simulink model "TEST3_Control_Simulink"  (R2025b)
settings: Solver=ode3  StartTime=0.0  StopTime=500  FixedStep=0.1  RelTol=1e-3
libraries: slpidlib x2
settings Model: Creator=daniel.camacho  LastModifiedBy=daniel.camacho

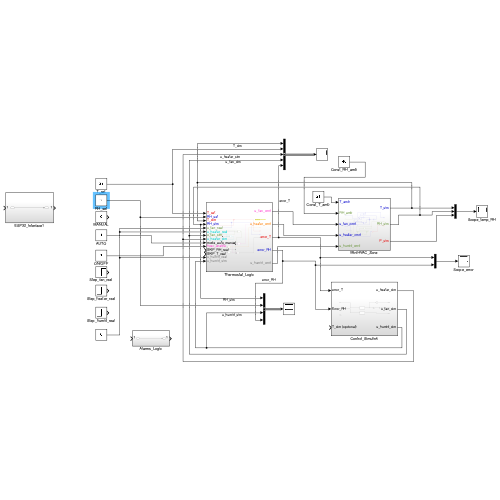
[thumbnail: Simulink's stored preview of the top-level diagram]
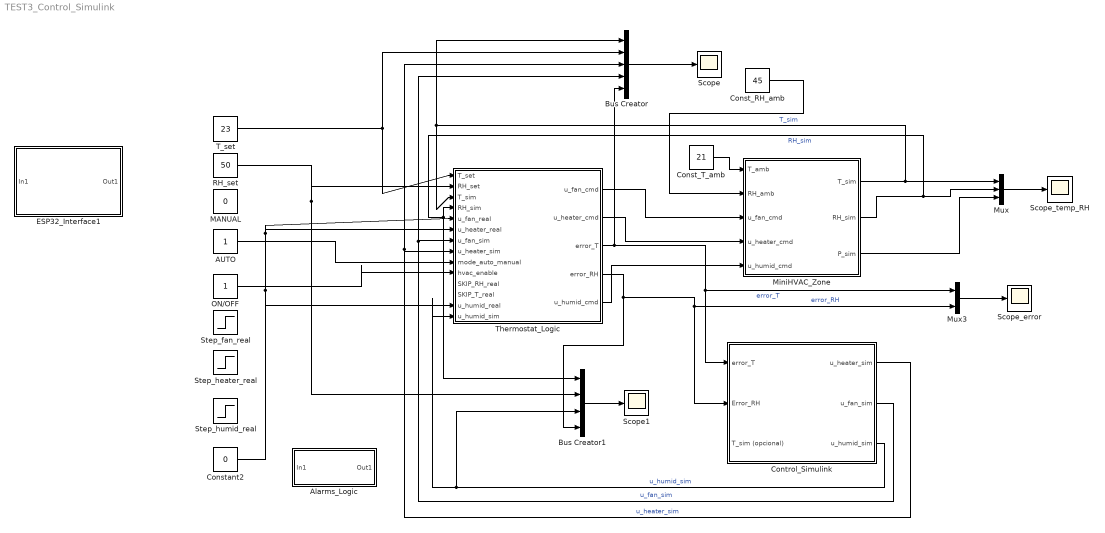
== system TEST3_Control_Simulink ==
  AUTO : Constant
  Alarms_Logic : Subsystem
  Bus Creator : BusCreator  Inputs=5
  Bus Creator1 : BusCreator  Inputs=4
  Const_RH_amb : Constant  Value=45
  Const_T_amb : Constant  Value=21
  Constant2 : Constant  Value=0
  Control_Simulink : Subsystem
  ESP32_Interface1 : Subsystem
  MANUAL : Constant  Value=0
  MiniHVAC_Zone : Subsystem
  Mux : Mux  Inputs=3
  Mux3 : Mux  Inputs=2
  ON/OFF : Constant
  RH_set : Constant  Value=50
  Scope : Scope
      settings: ActiveDisplayYMinimum=-7.8749999999999991  ActiveDisplayYMaximum=30.875  DataLoggingVariableName=ScopeData2
  Scope1 : Scope
      settings: ActiveDisplayYMinimum=-3.7726610995942522  ActiveDisplayYMaximum=85.751334887185152
  Scope_error : Scope
      settings: ActiveDisplayYMinimum=-12.97347055879947  ActiveDisplayYMaximum=6.9970522843110521  DataLoggingVariableName=ScopeData4
  Scope_temp_RH : Scope
      settings: ActiveDisplayYMinimum=-1  ActiveDisplayYMaximum=1
  Step_fan_real : Step  Time=10  SampleTime=0
  Step_heater_real : Step  Time=20  SampleTime=0
  Step_humid_real : Step  Time=10  SampleTime=0
  T_set : Constant  Value=23
  Thermostat_Logic : Subsystem
  wires:
  RH_set/1 -> Thermostat_Logic/2(RH_set), Bus Creator1/2
  ON/OFF/1 -> Thermostat_Logic/10(hvac_enable)
  Constant2/1 -> Thermostat_Logic/13(u_humid_real), Thermostat_Logic/6(u_heater_real), Thermostat_Logic/5(u_fan_real)
  MiniHVAC_Zone/2(RH_sim) -> Mux/2, Bus Creator1/1, Thermostat_Logic/4(RH_sim)  "RH_sim"
  Thermostat_Logic/1(u_fan_cmd) -> MiniHVAC_Zone/3(u_fan_cmd)
  Thermostat_Logic/2(u_heater_cmd) -> MiniHVAC_Zone/4(u_heater_cmd)
  Const_T_amb/1 -> MiniHVAC_Zone/1(T_amb)
  Const_RH_amb/1 -> MiniHVAC_Zone/2(RH_amb)
  Mux/1 -> Scope_temp_RH/1
  MiniHVAC_Zone/3(P_sim) -> Mux/3
  Mux3/1 -> Scope_error/1
  Thermostat_Logic/4(error_RH) -> Bus Creator1/4, Mux3/2, Control_Simulink/2(Error_RH)  "error_RH"
  Thermostat_Logic/5(u_humid_cmd) -> MiniHVAC_Zone/5(u_humid_cmd)
  T_set/1 -> Thermostat_Logic/1(T_set), Bus Creator/2
  Thermostat_Logic/3(error_T) -> Mux3/1, Control_Simulink/1(error_T), Bus Creator/5  "error_T"
  MiniHVAC_Zone/1(T_sim) -> Mux/1, Bus Creator/1, Thermostat_Logic/3(T_sim)  "T_sim"
  Control_Simulink/2(u_fan_sim) -> Bus Creator/4, Thermostat_Logic/7(u_fan_sim)  "u_fan_sim"
  Control_Simulink/1(u_heater_sim) -> Bus Creator/3, Thermostat_Logic/8(u_heater_sim)  "u_heater_sim"
  Bus Creator/1 -> Scope/1
  AUTO/1 -> Thermostat_Logic/9(mode_auto_manual)
  Bus Creator1/1 -> Scope1/1
  Control_Simulink/3(u_humid_sim) -> Bus Creator1/3, Thermostat_Logic/14(u_humid_sim)  "u_humid_sim"

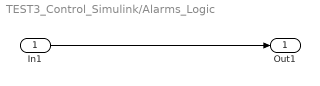
== system TEST3_Control_Simulink/Alarms_Logic ==
  In1 : Inport
  Out1 : Outport
  wires:
  In1/1 -> Out1/1

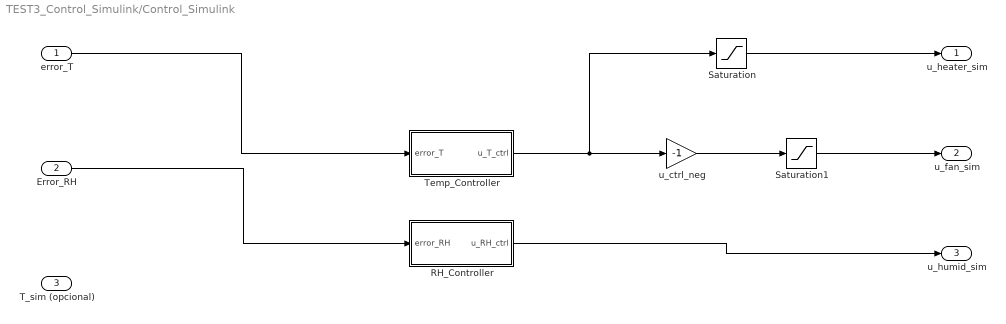
== system TEST3_Control_Simulink/Control_Simulink ==
  error_T : Inport
  Error_RH : Inport  Port=2
  T_sim (opcional) : Inport  Port=3
  RH_Controller : Subsystem
  Saturation : Saturate  UpperLimit=1  LowerLimit=0
  Saturation1 : Saturate  UpperLimit=1  LowerLimit=0
  Temp_Controller : Subsystem
  u_ctrl_neg : Gain  Gain=-1
  u_heater_sim : Outport
  u_fan_sim : Outport  Port=2
  u_humid_sim : Outport  Port=3
  wires:
  Temp_Controller/1(u_T_ctrl) -> u_ctrl_neg/1, Saturation/1
  Saturation/1 -> u_heater_sim/1
  u_ctrl_neg/1 -> Saturation1/1
  Saturation1/1 -> u_fan_sim/1
  error_T/1 -> Temp_Controller/1(error_T)
  Error_RH/1 -> RH_Controller/1(error_RH)
  RH_Controller/1(u_RH_ctrl) -> u_humid_sim/1

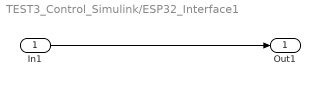
== system TEST3_Control_Simulink/ESP32_Interface1 ==
  In1 : Inport
  Out1 : Outport
  wires:
  In1/1 -> Out1/1

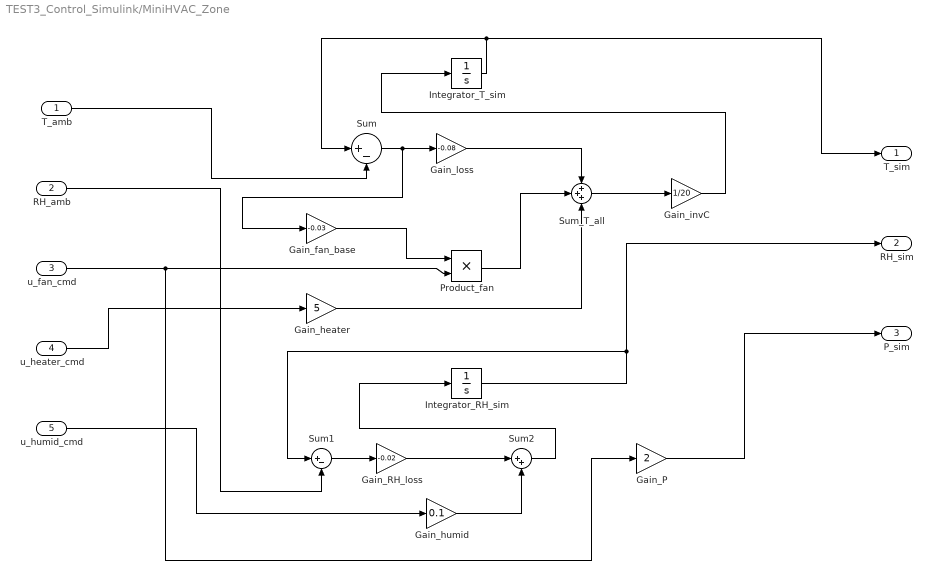
== system TEST3_Control_Simulink/MiniHVAC_Zone ==
  T_amb : Inport
  RH_amb : Inport  Port=2
  u_fan_cmd : Inport  Port=3
  u_heater_cmd : Inport  Port=4
  u_humid_cmd : Inport  Port=5
  Gain_P : Gain  Gain=2
  Gain_RH_loss : Gain  Gain=-0.02
  Gain_fan_base : Gain  Gain=-0.03
  Gain_heater : Gain  Gain=5
  Gain_humid : Gain  Gain=0.1
  Gain_invC : Gain  Gain=1/20
  Gain_loss : Gain  Gain=-0.08
  Integrator_RH_sim : Integrator  InitialCondition=45
  Integrator_T_sim : Integrator  InitialCondition=27
  Product_fan : Product
  Sum : Sum  Inputs=|+-
  Sum1 : Sum  Inputs=|+-
  Sum2 : Sum  Inputs=|++
  Sum_T_all : Sum  Inputs=+++
  T_sim : Outport
  RH_sim : Outport  Port=2
  P_sim : Outport  Port=3
  wires:
  Integrator_T_sim/1 -> T_sim/1, Sum/1
  T_amb/1 -> Sum/2
  Gain_fan_base/1 -> Product_fan/1
  u_fan_cmd/1 -> Gain_P/1, Product_fan/2
  u_heater_cmd/1 -> Gain_heater/1
  Sum/1 -> Gain_loss/1, Gain_fan_base/1
  Gain_loss/1 -> Sum_T_all/1
  Product_fan/1 -> Sum_T_all/2
  Gain_heater/1 -> Sum_T_all/3
  Sum_T_all/1 -> Gain_invC/1
  Gain_invC/1 -> Integrator_T_sim/1
  Integrator_RH_sim/1 -> RH_sim/1, Sum1/1
  RH_amb/1 -> Sum1/2
  Sum1/1 -> Gain_RH_loss/1
  u_humid_cmd/1 -> Gain_humid/1
  Gain_RH_loss/1 -> Sum2/1
  Gain_humid/1 -> Sum2/2
  Sum2/1 -> Integrator_RH_sim/1
  Gain_P/1 -> P_sim/1

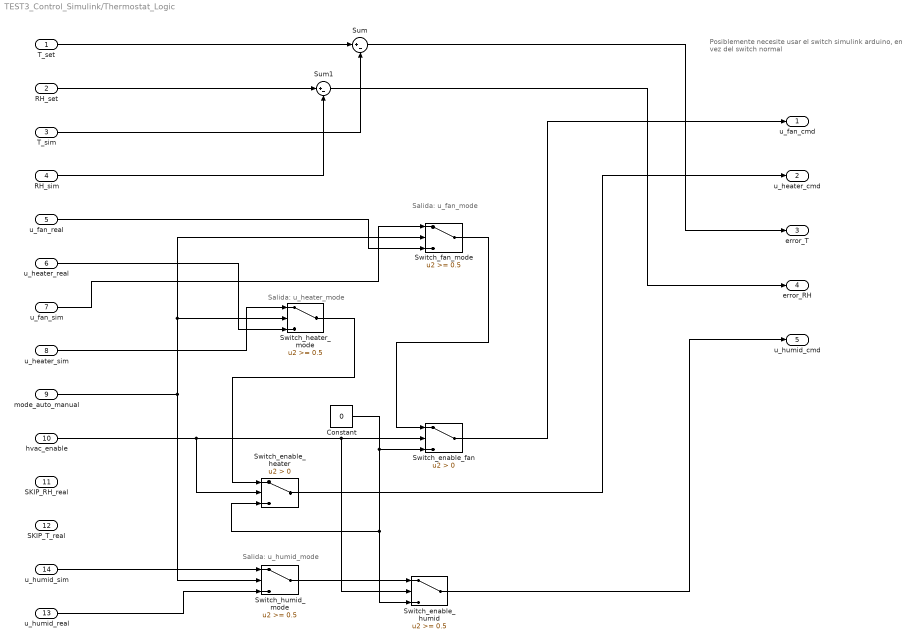
== system TEST3_Control_Simulink/Thermostat_Logic ==
  note: Salida: u_fan_mode
  note: Posiblemente necesite usar el switch simulink arduino,
      | en vez del switch normal
  note: Salida: u_heater_mode
  note: Salida: u_humid_mode
  T_set : Inport
  RH_set : Inport  Port=2
  T_sim : Inport  Port=3
  RH_sim : Inport  Port=4
  u_fan_real : Inport  Port=5
  u_heater_real : Inport  Port=6
  u_fan_sim : Inport  Port=7
  u_heater_sim : Inport  Port=8
  mode_auto_manual : Inport  Port=9
  hvac_enable : Inport  Port=10
  SKIP_RH_real : Inport  Port=11
  SKIP_T_real : Inport  Port=12
  u_humid_real : Inport  Port=13
  u_humid_sim : Inport  Port=14
  Constant : Constant  Value=0
  Sum : Sum  Inputs=|+-
  Sum1 : Sum  Inputs=|+-
  Switch_enable_fan : Switch  Criteria=u2 > Threshold  SaturateOnIntegerOverflow=off  InputSameDT=off
  Switch_enable_heater : Switch  Criteria=u2 > Threshold  SaturateOnIntegerOverflow=off  InputSameDT=off
  Switch_enable_humid : Switch  Threshold=0.5  SaturateOnIntegerOverflow=off  InputSameDT=off
  Switch_fan_mode : Switch  Threshold=0.5  SaturateOnIntegerOverflow=off  InputSameDT=off
  Switch_heater_mode : Switch  Threshold=0.5  OutMin=0  OutMax=1  SaturateOnIntegerOverflow=off  InputSameDT=off
  Switch_humid_mode : Switch  Threshold=0.5  SaturateOnIntegerOverflow=off  InputSameDT=off
  u_fan_cmd : Outport
  u_heater_cmd : Outport  Port=2
  error_T : Outport  Port=3
  error_RH : Outport  Port=4
  u_humid_cmd : Outport  Port=5
  wires:
  T_set/1 -> Sum/1
  T_sim/1 -> Sum/2
  Sum/1 -> error_T/1
  RH_set/1 -> Sum1/1
  RH_sim/1 -> Sum1/2
  Sum1/1 -> error_RH/1
  mode_auto_manual/1 -> Switch_heater_mode/2, Switch_fan_mode/2, Switch_humid_mode/2
  Constant/1 -> Switch_enable_fan/3, Switch_enable_humid/3, Switch_enable_heater/3
  hvac_enable/1 -> Switch_enable_fan/2, Switch_enable_humid/2, Switch_enable_heater/2
  Switch_enable_fan/1 -> u_fan_cmd/1
  Switch_enable_heater/1 -> u_heater_cmd/1
  u_fan_real/1 -> Switch_fan_mode/3
  u_fan_sim/1 -> Switch_fan_mode/1
  u_heater_sim/1 -> Switch_heater_mode/1
  u_heater_real/1 -> Switch_heater_mode/3
  Switch_fan_mode/1 -> Switch_enable_fan/1
  Switch_heater_mode/1 -> Switch_enable_heater/1
  u_humid_sim/1 -> Switch_humid_mode/1
  u_humid_real/1 -> Switch_humid_mode/3
  Switch_humid_mode/1 -> Switch_enable_humid/1
  Switch_enable_humid/1 -> u_humid_cmd/1

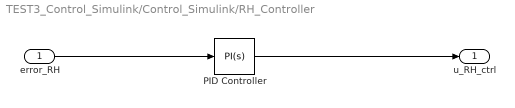
== system TEST3_Control_Simulink/Control_Simulink/RH_Controller ==
  error_RH : Inport
  PID Controller : slpidlib/PID Controller  Controller=PI  Form=Parallel  TimeDomain=Continuous-time  UseExternalTs=off  SampleTime=-1  IntegratorMethod=Forward Euler  FilterMethod=Forward Euler  ControllerParametersSource=internal  P=0.5  I=0.01  UseKiTs=off  D=0  UseExternalDerivativeSource=off  N=100  UseFilter=on  TunerSelectOption=Transfer Function Based (PID Tuner App)  InitialConditionSource=internal  InitialConditionForIntegrator=0  InitialConditionForFilter=0  DifferentiatorICPrevScaledInput=0  ExternalReset=none  TrackingMode=off  Kt=1  LimitOutput=on  SatLimitsSource=internal  UpperSaturationLimit=1  LowerSaturationLimit=0  LinearizeAsGain=on  AntiWindupMode=back-calculation  Kb=1  LimitIntegrator=off  UpperIntegratorSaturationLimit=inf  LowerIntegratorSaturationLimit=-inf  POutMin=[]  POutMax=[]  IOutMin=[]  IOutMax=[]  DOutMin=[]  DOutMax=[]  NOutMin=[]  NOutMax=[]  SumOutMin=[]  SumOutMax=[]  SaturationOutMin=[]  SaturationOutMax=[]  PParamMin=[]  PParamMax=[]  IParamMin=[]  IParamMax=[]  DParamMin=[]  DParamMax=[]  NParamMin=[]  NParamMax=[]  KbParamMin=[]  KbParamMax=[]  KtParamMin=[]  KtParamMax=[]  KbOutMin=[]  KbOutMax=[]  KtOutMin=[]  KtOutMax=[]  IntegratorOutMin=[]  IntegratorOutMax=[]  FilterOutMin=[]  FilterOutMax=[]  SumI1OutMin=[]  SumI1OutMax=[]  SumI2OutMin=[]  SumI2OutMax=[]  SumI3OutMin=[]  SumI3OutMax=[]  SumI4OutMin=[]  SumI4OutMax=[]  SumDOutMin=[]  SumDOutMax=[]  DifferentiatorOutMin=[]  DifferentiatorOutMax=[]  FilterDiffOutCoefMin=[]  FilterDiffOutCoefMax=[]  ReciprocalOutMin=[]  ReciprocalOutMax=[]  SumDenOutMin=[]  SumDenOutMax=[]  SumNumOutMin=[]  SumNumOutMax=[]  DivideOutMin=[]  DivideOutMax=[]  UdiffTsProdOutMin=[]  UdiffTsProdOutMax=[]  NTsProdOutMin=[]  NTsProdOutMax=[]  UintegralTsProdOutMin=[]  UintegralTsProdOutMax=[]  UngainTsProdOutMin=[]  UngainTsProdOutMax=[]  ClampingZeroOutDataTypeStr=Inherit: Inherit via back propagation  ClampingZeroOutMin=[]  ClampingZeroOutMax=[]  FilterDenConstantOutDataTypeStr=Inherit: Inherit via back propagation  FilterDenConstantOutMin=[]  FilterDenConstantOutMax=[]  PCopyOutDataTypeStr=Inherit: Inherit via back propagation  PCopyOutMin=[]  PCopyOutMax=[]  NCopyOutDataTypeStr=Inherit: Inherit via back propagation  NCopyOutMin=[]  NCopyOutMax=[]  IntegratorContinuousStateAttributes=''  IntegratorStateMustResolveToSignalObject=off  IntegratorRTWStateStorageClass=Auto  FilterContinuousStateAttributes=''  FilterStateMustResolveToSignalObject=off  FilterRTWStateStorageClass=Auto  ParallelPVariant=InternalParameters  IdealPVariant=Disabled  IVariant=InternalParameters  DVariant=Disabled  IntegratorVariant=Continuous  SatVariant=Enabled  AWVariant=BackCalculation  PCopyVariant=Disabled  TRVariant=Disabled  FdbkBlocksVariant=Forward  IdealPFdbkVariant=Disabled  SatFdbkVariant=Disabled  DerivativeFilterVariant=Disabled  NVariant=Disabled  NCopyVariant=Disabled_SignalSpec  FilterICVariant=Disabled  IntegratorICVariant=InternalICs  ExternalResetVariant=Disabled  TRSumVariant=Passthrough  SumFdbkVariant=Disabled  SumVariant=Sum_PI  TsampFilterVariant=InternalTs  TsampNgainVariant=Passthrough  TsampIntegralVariant=Disabled_SignalSpec  ExternalSaturationOutDataTypeStr=Inherit: Same as second input  DerivativeSourceVariant=Disabled  PreIntVariant=InternalPreInt
  u_RH_ctrl : Outport
  wires:
  error_RH/1 -> PID Controller/1
  PID Controller/1 -> u_RH_ctrl/1

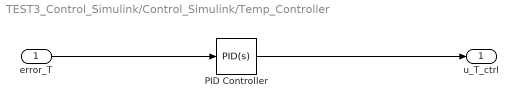
== system TEST3_Control_Simulink/Control_Simulink/Temp_Controller ==
  error_T : Inport
  PID Controller : slpidlib/PID Controller  Controller=PID  Form=Parallel  TimeDomain=Continuous-time  UseExternalTs=off  SampleTime=-1  IntegratorMethod=Forward Euler  FilterMethod=Forward Euler  ControllerParametersSource=internal  P=0.5  I=0.01  UseKiTs=off  D=0  UseExternalDerivativeSource=off  N=100  UseFilter=on  TunerSelectOption=Transfer Function Based (PID Tuner App)  InitialConditionSource=internal  InitialConditionForIntegrator=0  InitialConditionForFilter=0  DifferentiatorICPrevScaledInput=0  ExternalReset=none  TrackingMode=off  Kt=1  LimitOutput=on  SatLimitsSource=internal  UpperSaturationLimit=1  LowerSaturationLimit=-1  LinearizeAsGain=on  AntiWindupMode=back-calculation  Kb=1  LimitIntegrator=off  UpperIntegratorSaturationLimit=inf  LowerIntegratorSaturationLimit=-inf  POutMin=[]  POutMax=[]  IOutMin=[]  IOutMax=[]  DOutMin=[]  DOutMax=[]  NOutMin=[]  NOutMax=[]  SumOutMin=[]  SumOutMax=[]  SaturationOutMin=[]  SaturationOutMax=[]  PParamMin=[]  PParamMax=[]  IParamMin=[]  IParamMax=[]  DParamMin=[]  DParamMax=[]  NParamMin=[]  NParamMax=[]  KbParamMin=[]  KbParamMax=[]  KtParamMin=[]  KtParamMax=[]  KbOutMin=[]  KbOutMax=[]  KtOutMin=[]  KtOutMax=[]  IntegratorOutMin=[]  IntegratorOutMax=[]  FilterOutMin=[]  FilterOutMax=[]  SumI1OutMin=[]  SumI1OutMax=[]  SumI2OutMin=[]  SumI2OutMax=[]  SumI3OutMin=[]  SumI3OutMax=[]  SumI4OutMin=[]  SumI4OutMax=[]  SumDOutMin=[]  SumDOutMax=[]  DifferentiatorOutMin=[]  DifferentiatorOutMax=[]  FilterDiffOutCoefMin=[]  FilterDiffOutCoefMax=[]  ReciprocalOutMin=[]  ReciprocalOutMax=[]  SumDenOutMin=[]  SumDenOutMax=[]  SumNumOutMin=[]  SumNumOutMax=[]  DivideOutMin=[]  DivideOutMax=[]  UdiffTsProdOutMin=[]  UdiffTsProdOutMax=[]  NTsProdOutMin=[]  NTsProdOutMax=[]  UintegralTsProdOutMin=[]  UintegralTsProdOutMax=[]  UngainTsProdOutMin=[]  UngainTsProdOutMax=[]  ClampingZeroOutDataTypeStr=Inherit: Inherit via back propagation  ClampingZeroOutMin=[]  ClampingZeroOutMax=[]  FilterDenConstantOutDataTypeStr=Inherit: Inherit via back propagation  FilterDenConstantOutMin=[]  FilterDenConstantOutMax=[]  PCopyOutDataTypeStr=Inherit: Inherit via back propagation  PCopyOutMin=[]  PCopyOutMax=[]  NCopyOutDataTypeStr=Inherit: Inherit via back propagation  NCopyOutMin=[]  NCopyOutMax=[]  IntegratorContinuousStateAttributes=''  IntegratorStateMustResolveToSignalObject=off  IntegratorRTWStateStorageClass=Auto  FilterContinuousStateAttributes=''  FilterStateMustResolveToSignalObject=off  FilterRTWStateStorageClass=Auto  ParallelPVariant=InternalParameters  IdealPVariant=Disabled  IVariant=InternalParameters  DVariant=InternalParameters  IntegratorVariant=Continuous  SatVariant=Enabled  AWVariant=BackCalculation  PCopyVariant=Disabled  TRVariant=Disabled  FdbkBlocksVariant=Forward  IdealPFdbkVariant=Disabled  SatFdbkVariant=Disabled  DerivativeFilterVariant=ContFilter  NVariant=InternalParameters  NCopyVariant=Disabled  FilterICVariant=InternalICsFilter  IntegratorICVariant=InternalICs  ExternalResetVariant=Disabled  TRSumVariant=Passthrough  SumFdbkVariant=Disabled  SumVariant=Sum_PID  TsampFilterVariant=InternalTs  TsampNgainVariant=Passthrough  TsampIntegralVariant=Disabled_SignalSpec  ExternalSaturationOutDataTypeStr=Inherit: Same as second input  DerivativeSourceVariant=ErrorSignal  PreIntVariant=InternalPreInt
  u_T_ctrl : Outport
  wires:
  error_T/1 -> PID Controller/1
  PID Controller/1 -> u_T_ctrl/1
